simulink model "circ_mo"  (R2018b)
settings: Solver=VariableStepAuto  StartTime=0.0  StopTime=5  RelTol=1e-9
libraries: shared6dof x1, aerolibanim x1, vrlib x1, dspmtrx3 x1
settings Model: Creator=mendicantbias  LastModifiedBy=mendicantbias

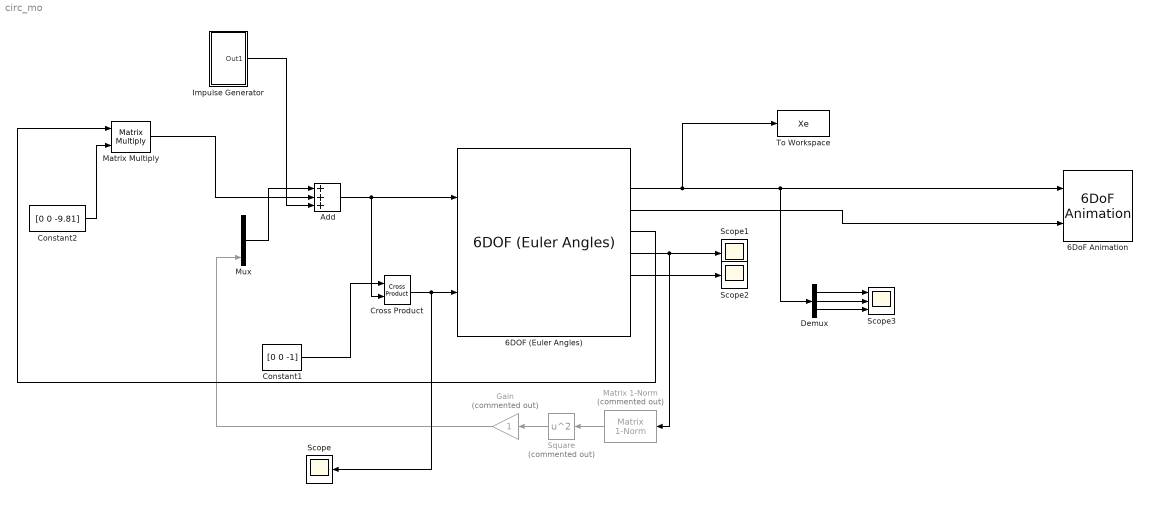
== system circ_mo ==
  6DOF (Euler Angles) : shared6dof/6DOF (Euler Angles)  units=Metric (MKS)  mtype=Fixed  rep=Quaternion  xme_0=[0 0 0]  Vm_0=[0 0 0]  eul_0=[0 0 0]  pm_0=[0 0 0]  mass_0=1.0  mass_e=0.5  mass_f=2.0  inertia=eye(3)  inertia_e=eye(3)  inertia_f=2*eye(3)  k_quat=1.0  vre_flag=on  abi_flag=off  aMode=0  xme_statename=''  Vm_statename=''  eul_statename=''  quat_statename=''  pm_statename=''  mass_statename=''
      settings: SourceProductBaseCode=AE
  6DoF Animation : aerolibanim/6DoF Animation  u1=[-5 5 -5 5 -5 5]  u2=0.1  u3=0.1  u4=[4000 0 -5000]  u5=Fly alongside  u6=[5 5 5]  u7=10  u8=on
      settings: SourceProductName=Aerospace Blockset
  Add : Sum  Inputs=+++
  Constant1 : Constant  Value=[0 0 -1]
  Constant2 : Constant  Value=[0 0 -9.81]
  Cross Product : vrlib/Utilities/Cross Product
      settings: SourceProductBaseCode=VR
  Demux : Demux  Outputs=3
  Gain : Gain  Commented=on
  Impulse Generator : Subsystem
  Matrix 1-Norm : dspmtrx3/Matrix  1-Norm  Commented=on  roundingMode=Floor  overflowMode=off  outputDataTypeStr=Inherit: Same as accumulator  outputMin=[]  outputMax=[]  outputLastDataTypeStr=Inherit: Same as accumulator
      settings: SourceProductName=DSP System Toolbox  SourceProductBaseCode=DS
  Matrix Multiply : Product  Multiplication=Matrix(*)
  Mux : Mux  Inputs=3
  Scope : Scope
  Scope1 : Scope
  Scope2 : Scope
  Scope3 : Scope  NumInputPorts=3
  Square : Math  Commented=on  Operator=square  SaturateOnIntegerOverflow=on
  To Workspace : ToWorkspace  VariableName=Xe  SaveFormat=Timeseries  SampleTime=-1
  wires:
  6DOF (Euler Angles)/2 -> To Workspace/1, Demux/1, 6DoF Animation/1
  6DOF (Euler Angles)/3 -> 6DoF Animation/2
  Matrix 1-Norm/1 -> Square/1
  Square/1 -> Gain/1
  6DOF (Euler Angles)/5 -> Scope1/1, Matrix 1-Norm/1
  Add/1 -> Cross Product/2, 6DOF (Euler Angles)/1
  Constant1/1 -> Cross Product/1
  Gain/1 -> Mux/3
  Cross Product/1 -> 6DOF (Euler Angles)/2, Scope/1
  6DOF (Euler Angles)/6 -> Scope2/1
  Demux/3 -> Scope3/3
  Demux/2 -> Scope3/2
  Demux/1 -> Scope3/1
  Mux/1 -> Add/1
  Constant2/1 -> Matrix Multiply/2
  6DOF (Euler Angles)/4 -> Matrix Multiply/1
  Impulse Generator/1(Out1) -> Add/3
  Matrix Multiply/1 -> Add/2

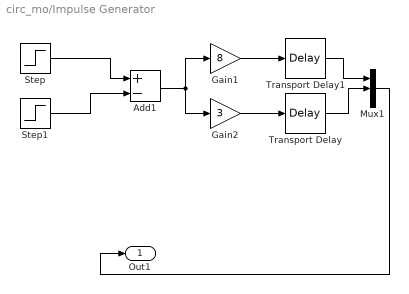
== system circ_mo/Impulse Generator ==
  Add1 : Sum  Inputs=+-
  Gain1 : Gain  Gain=8
  Gain2 : Gain  Gain=3
  Mux1 : Mux  Inputs=3
  Step : Step  SampleTime=0
  Step1 : Step  Time=1.2  SampleTime=0
  Transport Delay : TransportDelay  DelayTime=0
  Transport Delay1 : TransportDelay  DelayTime=0
  Out1 : Outport
  wires:
  Step/1 -> Add1/1
  Step1/1 -> Add1/2
  Gain1/1 -> Transport Delay1/1
  Transport Delay/1 -> Mux1/2
  Add1/1 -> Gain2/1, Gain1/1
  Mux1/1 -> Out1/1
  Transport Delay1/1 -> Mux1/1
  Gain2/1 -> Transport Delay/1
